simulink model "fuzzytfg1"  (R2020b)
settings: Solver=VariableStepAuto  StartTime=0.0  StopTime=20.0  RelTol=1e-3
libraries: fuzblock x1
settings Model: Creator=diosdado  LastModifiedBy=alumnoic03

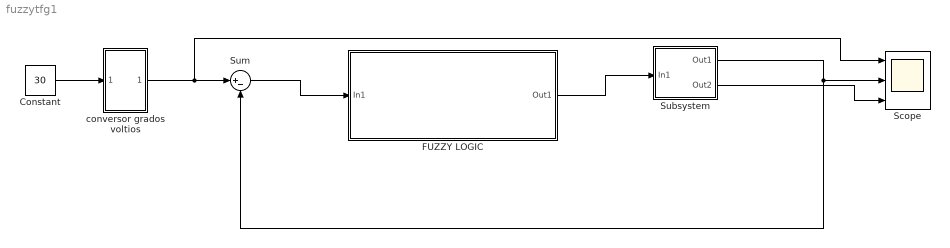
== system fuzzytfg1 ==
  Constant : Constant  Value=30
  FUZZY LOGIC : Subsystem
  Scope : Scope  NumInputPorts=3
  Subsystem : Subsystem
  Sum : Sum  Inputs=|+-
  "conversor grados voltios " : Subsystem  mask{a=4.95, b=0.869}
  wires:
  Constant/1 -> "conversor grados voltios "/1(In1)
  Subsystem/1(Out1) -> Sum/2, Scope/2
  Subsystem/2(Out2) -> Scope/3
  "conversor grados voltios "/1(Out1) -> Scope/1, Sum/1
  Sum/1 -> FUZZY LOGIC/1(In1)
  FUZZY LOGIC/1(Out1) -> Subsystem/1(In1)

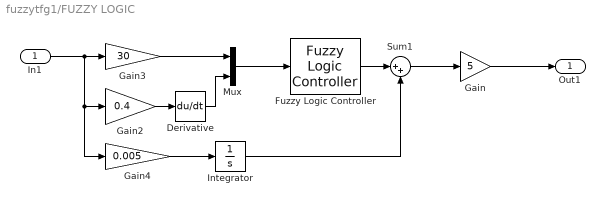
== system fuzzytfg1/FUZZY LOGIC ==
  In1 : Inport
  Derivative : Derivative
  Fuzzy Logic Controller : fuzblock/Fuzzy Logic  Controller  FIS='FUZZY3.fis'  OutputSampleNumber=101  DataType=double  FuzzifiedInputs=off  RuleFiringStrengths=off  RuleOutputs=off  AggregatedOutputs=off  SimulateUsing=Interpreted execution  OutOfRangeInputValueMessage=warning  NoRuleFiredMessage=warning  EmptyOutputFuzzySetMessage=warning
  Gain : Gain  Gain=5
  Gain2 : Gain  Gain=0.4
  Gain3 : Gain  Gain=30
  Gain4 : Gain  Gain=0.005
  Integrator : Integrator
  Mux : Mux  Inputs=2
  Sum1 : Sum  Inputs=|++
  Out1 : Outport
  wires:
  Derivative/1 -> Mux/2
  In1/1 -> Gain3/1, Gain2/1, Gain4/1
  Mux/1 -> Fuzzy Logic Controller/1
  Gain3/1 -> Mux/1
  Fuzzy Logic Controller/1 -> Sum1/1
  Gain2/1 -> Derivative/1
  Gain4/1 -> Integrator/1
  Integrator/1 -> Sum1/2
  Sum1/1 -> Gain/1
  Gain/1 -> Out1/1

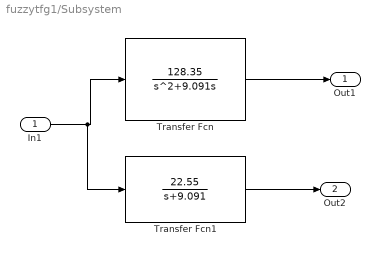
== system fuzzytfg1/Subsystem ==
  In1 : Inport
  Transfer Fcn : TransferFcn  Numerator=[128.35]  Denominator=[1 9.091 0]
  Transfer Fcn1 : TransferFcn  Numerator=[22.55]  Denominator=[1 9.091]
  Out1 : Outport
  Out2 : Outport  Port=2
  wires:
  In1/1 -> Transfer Fcn1/1, Transfer Fcn/1
  Transfer Fcn/1 -> Out1/1
  Transfer Fcn1/1 -> Out2/1

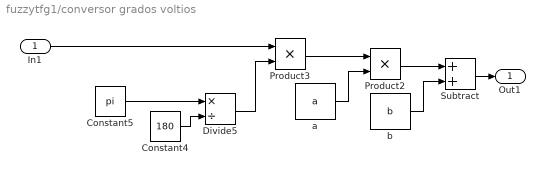
== system fuzzytfg1/conversor grados voltios  ==
  In1 : Inport
  Constant4 : Constant  Value=180
  Constant5 : Constant  Value=pi
  Divide5 : Product  Inputs=*/
  Product2 : Product
  Product3 : Product
  Subtract : Sum
  a : Constant  Value=a
  b : Constant  Value=b
  Out1 : Outport
  wires:
  b/1 -> Subtract/2
  Product3/1 -> Product2/1
  Constant4/1 -> Divide5/2
  In1/1 -> Product3/1
  Product2/1 -> Subtract/1
  a/1 -> Product2/2
  Constant5/1 -> Divide5/1
  Divide5/1 -> Product3/2
  Subtract/1 -> Out1/1
